simulink model "lab1"  (Simulink 4.00)
settings: Solver=ode45  StartTime=0.0  StopTime=10.0  RelTol=1e-3
settings Model: LastModifiedBy=daemok

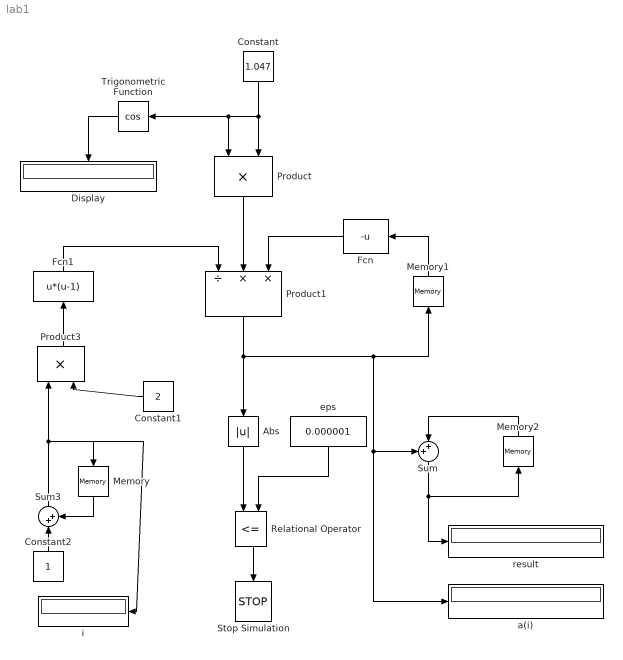
== system lab1 ==
  Abs : Abs  Orientation=down  SaturateOnIntegerOverflow=on
  Constant : Constant  Orientation=down  Value=1.047
  Constant1 : Constant  Orientation=left  Value=2
  Constant2 : Constant  Orientation=up  Value=1
  Display : Display
      settings: Orientation=down
  Fcn : Fcn  Orientation=left  Expr=-u
  Fcn1 : Fcn  Orientation=up  Expr=u*(u-1)
  Memory : Memory  Orientation=down  X0=0  InheritSampleTime=off
      settings: RTWStateStorageClass=Auto
  Memory1 : Memory  Orientation=up  X0=1  InheritSampleTime=off
      settings: RTWStateStorageClass=Auto
  Memory2 : Memory  Orientation=up  X0=1  InheritSampleTime=off
      settings: RTWStateStorageClass=Auto
  Product : Product  Orientation=down  Inputs=2  Multiplication=Element-wise(.*)  SaturateOnIntegerOverflow=on
  Product1 : Product  Orientation=down  Inputs=/**  Multiplication=Element-wise(.*)  SaturateOnIntegerOverflow=on
  Product3 : Product  Orientation=up  Inputs=2  Multiplication=Element-wise(.*)  SaturateOnIntegerOverflow=on
  Relational Operator : RelationalOperator  Orientation=down  Operator=<=
  Stop Simulation : Stop  Orientation=down
  Sum : Sum  Orientation=down  Inputs=++|  SaturateOnIntegerOverflow=on
  Sum3 : Sum  Orientation=up  Inputs=|++  SaturateOnIntegerOverflow=on
  Trigonometric Function : Trigonometry  Orientation=left  Operator=cos  OutputSignalType=auto
  a(i) : Display
  eps : Constant  Orientation=down  Value=0.000001
  i : Display
      settings: Format=short
  result : Display
  wires:
  Constant/1 -> Product/2, Trigonometric Function/1, Product/1
  Trigonometric Function/1 -> Display/1
  Product/1 -> Product1/2
  Product1/1 -> Abs/1, Memory1/1, a(i)/1, Sum/1
  Abs/1 -> Relational Operator/1
  eps/1 -> Relational Operator/2
  Relational Operator/1 -> Stop Simulation/1
  Fcn/1 -> Product1/3
  Memory1/1 -> Fcn/1
  Memory2/1 -> Sum/2
  Sum/1 -> Memory2/1, result/1
  Constant1/1 -> Product3/2
  Constant2/1 -> Sum3/1
  Sum3/1 -> Product3/1, Memory/1, i/1
  Memory/1 -> Sum3/2
  Fcn1/1 -> Product1/1
  Product3/1 -> Fcn1/1
